simulink model "SimulinkFile"  (R2024b)
settings: Solver=VariableStepAuto  StartTime=0.0  StopTime=30  RelTol=1e-3
settings Model: Creator=swam  LastModifiedBy=root

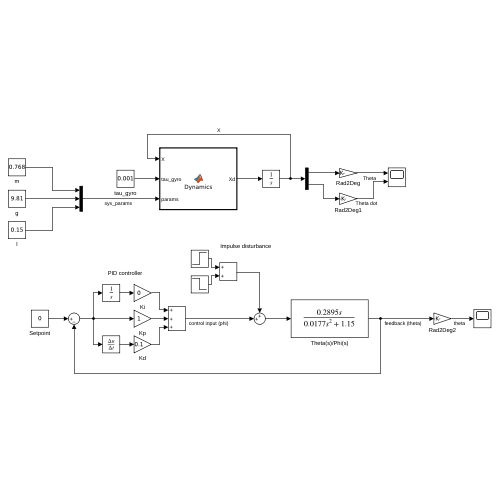
[thumbnail: Simulink's stored preview of the top-level diagram]
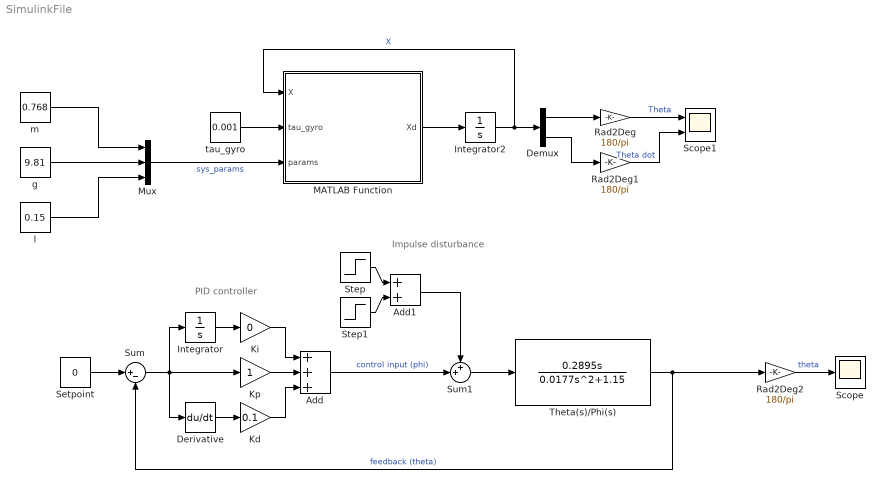
== system SimulinkFile ==
  note: Impulse disturbance
  note: PID controller
  Add : Sum  Inputs=+++
  Add1 : Sum
  Demux : Demux  Outputs=2
  Derivative : Derivative
  Integrator : Integrator
  Integrator2 : Integrator  InitialCondition=[20*pi/180;0]
  Kd : Gain  Gain=0.1
  Ki : Gain  Gain=0
  Kp : Gain
  MATLAB Function : MATLAB Function  TreatAsAtomicUnit=on
  Mux : Mux  Inputs=3
  Rad2Deg : Gain  Gain=180/pi
  Rad2Deg1 : Gain  Gain=180/pi
  Rad2Deg2 : Gain  Gain=180/pi
  Scope : Scope
  Scope1 : Scope  NumInputPorts=2
  Setpoint : Constant  Value=0
  Step : Step  Time=5  SampleTime=0.01
  Step1 : Step  Time=5.35  After=-1  SampleTime=0.01
  Sum : Sum  Inputs=|+-
  Sum1 : Sum  Inputs=++|
  Theta(s)/Phi(s) : TransferFcn  Numerator=[0.2895 0]  Denominator=[0.0177 0 1.15]
  g : Constant  Value=9.81  SampleTime=0.05
  l : Constant  Value=0.15  SampleTime=0.05
  m : Constant  Value=0.768  SampleTime=0.05
  tau_gyro : Constant  Value=0.001  SampleTime=0.05
  wires:
  m/1 -> Mux/1
  g/1 -> Mux/2
  l/1 -> Mux/3
  tau_gyro/1 -> MATLAB Function/2(tau_gyro)
  Mux/1 -> MATLAB Function/3(params)  "sys_params"
  MATLAB Function/1(Xd) -> Integrator2/1
  Integrator2/1 -> MATLAB Function/1(X), Demux/1  "X"
  Rad2Deg/1 -> Scope1/1  "Theta"
  Demux/1 -> Rad2Deg/1
  Demux/2 -> Rad2Deg1/1
  Rad2Deg1/1 -> Scope1/2  "Theta dot"
  Rad2Deg2/1 -> Scope/1  "theta"
  Setpoint/1 -> Sum/1
  Sum/1 -> Derivative/1, Kp/1, Integrator/1
  Integrator/1 -> Ki/1
  Derivative/1 -> Kd/1
  Kp/1 -> Add/2
  Ki/1 -> Add/1
  Kd/1 -> Add/3
  Theta(s)/Phi(s)/1 -> Rad2Deg2/1, Sum/2  "feedback (theta)"
  Add/1 -> Sum1/2  "control input (phi)"
  Add1/1 -> Sum1/1
  Step/1 -> Add1/1
  Step1/1 -> Add1/2
  Sum1/1 -> Theta(s)/Phi(s)/1

== matlab function SimulinkFile/MATLAB Function ==
  data: X input; Xd output; tau_gyro input; params input
function Xd = Dynamics(X, tau_gyro, params) %args : state vector, input torque, parametr values

%system parameters
m=params(1);
g=params(2);
l=params(3);
%I = m * l * l;

% state variables derivate vector
xd1 = X(2);
xd2 = (1/(m*l*l))*tau_gyro - (g/l)*(X(1)) ;
Xd = [xd1;xd2];
